simulink model "sliding"  (R2024a)
settings: Solver=FixedStepAuto  StartTime=0.0  StopTime=20  FixedStep=0.002  MaxStep=0.05  RelTol=1e-3
settings Model: Creator=Lenovo  LastModifiedBy=Lenovo
settings DebuggingCC: UnconnectedInputMsg=warning  UnconnectedOutputMsg=warning  UnconnectedLineMsg=warning
settings ModelReferenceCC: EnableRefExpFcnMdlSchedulingChecks=on
settings RTWCC: GPUComputeCapability=3.5  DLArmComputeVersion=19.05

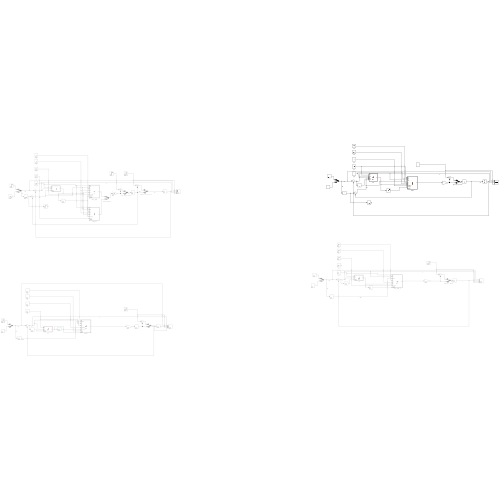
[thumbnail: Simulink's stored preview of the top-level diagram]
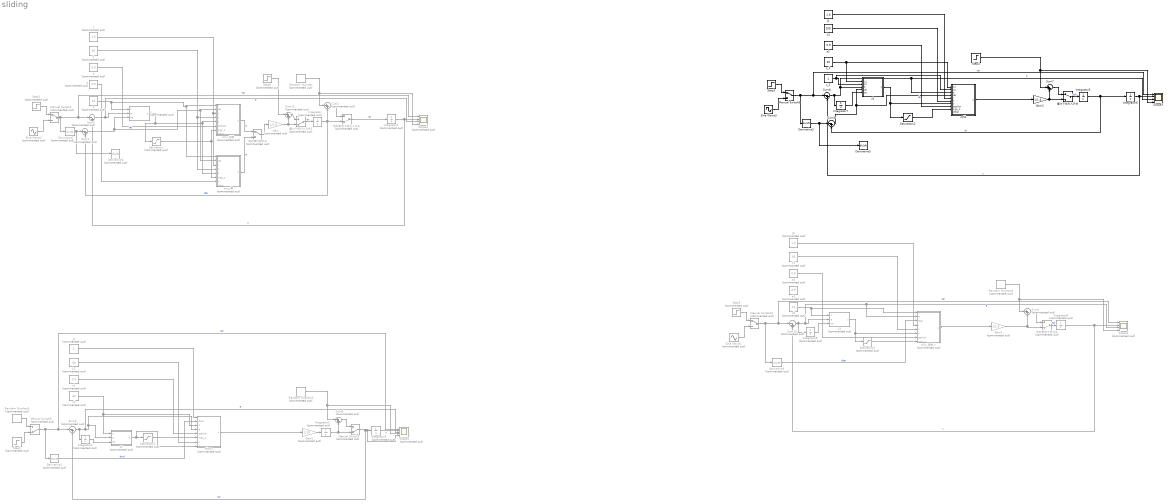
== system sliding ==
  Derivative{1..2,4,6} (4 alike) : Derivative  Commented=on
  Derivative3 : Derivative
  Derivative5 : Derivative
  Gain : Gain  Commented=on  Gain=1/1.6
  Gain1 : Gain  Commented=on  Gain=1/10
  Gain2 : Gain  Gain=1/1.6
  Gain3 : Gain  Commented=on  Gain=1/1.6
  Integrator{,1..4,8..9} (7 alike) : Integrator  Commented=on
  Integrator5 : Integrator
  Integrator6 : Integrator
  Integrator7 : Integrator
  J : Constant  Commented=on  Value=1.6
  J1 : Constant  Commented=on
  J2 : Constant  Value=1.6
  J3 : Constant  Commented=on  Value=1.6
  Manual Switch10 : ManualSwitch  Commented=on
  Manual Switch2 : ManualSwitch  Commented=on
  Manual Switch5 : ManualSwitch  Commented=on  CurrentSetting=0
  Manual Switch6 : ManualSwitch  Commented=on  CurrentSetting=0
  Manual Switch8 : ManualSwitch
  Random Number : RandomNumber  Commented=on  Seed=1  SampleTime=1
  Random Number2 : RandomNumber  Commented=on  Seed=1  SampleTime=1
  Random Number3 : RandomNumber  Commented=on  Variance=2  SampleTime=0.006
  Random Number4 : RandomNumber  Commented=on  Seed=1  SampleTime=1
  Saturation : Saturate  Commented=on  UpperLimit=0  LowerLimit=0
  Saturation1 : Saturate  Commented=on  UpperLimit=0  LowerLimit=0
  Saturation2 : Saturate  UpperLimit=0  LowerLimit=0
  Saturation3 : Saturate  Commented=on  UpperLimit=0  LowerLimit=0
  Scope1 : Scope  Commented=on  NumInputPorts=4
  Scope2 : Scope  Commented=on  NumInputPorts=5
  Scope3 : Scope  NumInputPorts=4
  Scope4 : Scope  Commented=on  NumInputPorts=4
  Sine Wave1 : Sin  Commented=on  Frequency=1*pi  SampleTime=0
  Sine Wave2 : Sin  Commented=on  Frequency=1*pi  SampleTime=0
  Sine Wave3 : Sin  Frequency=100*pi  SampleTime=0
  Step1 : Step  Commented=on  After=10  SampleTime=0
  Step2 : Step  Commented=on  SampleTime=0
  Step3 : Step  SampleTime=0
  Step4 : Step  After=50  SampleTime=0
  Step5 : Step  Commented=on  SampleTime=0
  Step6 : Step  Commented=on  After=50  SampleTime=0
  Sum{1..2,5,11} (4 alike) : Sum  Commented=on  Inputs=|++
  Sum{3..4,6,10} (4 alike) : Sum  Commented=on  Inputs=|-+
  Sum7 : Sum  Inputs=|++
  Sum8 : Sum  Inputs=|-+
  Sum9 : Sum  Inputs=|-+
  a : Constant  Commented=on  Value=0.9
  a1 : Constant  Commented=on  Value=0.9
  c : Constant  Commented=on  Value=13
  c1 : Constant  Commented=on  Value=40
  c2 : Constant  Commented=on  Value=13
  c_1 : Constant  Value=20
  c_2 : Constant
  ctrl4 : MATLAB Function  TreatAsAtomicUnit=on
  k : Constant  Commented=on  Value=95
  k1 : Constant  Commented=on  Value=60
  k2 : Constant  Value=200
  k3 : Constant  Commented=on  Value=95
  s : MATLAB Function  Commented=on  TreatAsAtomicUnit=on
  s1 : MATLAB Function  Commented=on  TreatAsAtomicUnit=on
  s2 : MATLAB Function  TreatAsAtomicUnit=on
  s3 : MATLAB Function  Commented=on  TreatAsAtomicUnit=on
  smc_幂 : MATLAB Function  Commented=on  TreatAsAtomicUnit=on
  smc_指数 : MATLAB Function  Commented=on  TreatAsAtomicUnit=on
  smc_指数_v : MATLAB Function  Commented=on  TreatAsAtomicUnit=on
  tfsmc : MATLAB Function  Commented=on  TreatAsAtomicUnit=on
  ε : Constant  Commented=on  Value=0.9
  ε1 : Constant  Commented=on  Value=0.5
  ε2 : Constant  Value=0.9
  ε3 : Constant  Commented=on  Value=0.8
  电机电流干扰开关 : ManualSwitch  Commented=on  CurrentSetting=0
  电机电流干扰引入开关 : ManualSwitch  Commented=on  CurrentSetting=0
  趋近律切换开关 : ManualSwitch  Commented=on
  重力干扰引入开关 : ManualSwitch
  重力干扰引入开关1 : ManualSwitch  Commented=on  CurrentSetting=0
  wires:
  c/1 -> smc_幂/1(c), smc_指数/1(c), s/1(c)
  Sum4/1 -> smc_幂/2(de), smc_指数/2(de), s/3(de)  "de"
  s/1(s) -> smc_幂/5(s), smc_指数/5(s), Saturation/1
  k/1 -> smc_幂/4(k), smc_指数/4(k)
  Step2/1 -> Manual Switch2/1
  Sine Wave2/1 -> Manual Switch2/2
  Integrator1/1 -> Scope1/2, Sum3/2  "x"
  J/1 -> smc_幂/3(J), smc_指数/3(J)
  ε/1 -> smc_指数/6(epsilon)
  Manual Switch2/1 -> Scope1/1, Sum3/1, Derivative2/1  "tar"
  Sum3/1 -> Scope1/3, s/2(e)  "e"
  Random Number/1 -> Scope1/4, Sum2/1
  Sum2/1 -> 电机电流干扰引入开关/1
  Integrator/1 -> Sum2/2, Sum4/2, 电机电流干扰引入开关/2  "ddx"
  smc_指数/1(u) -> 趋近律切换开关/1  "e"
  smc_幂/1(u) -> 趋近律切换开关/2  "e"
  趋近律切换开关/1 -> Gain/1
  Saturation/1 -> smc_指数/7(sign_s), smc_幂/6(sign_s)
  a/1 -> smc_幂/7(a)
  Sum5/1 -> Manual Switch5/1
  Random Number3/1 -> Manual Switch6/1
  Manual Switch6/1 -> Scope2/1, Sum6/1, Derivative1/1  "tar"
  Step1/1 -> Manual Switch6/2
  Sum6/1 -> Integrator4/1, Scope2/3, tfsmc/4(e), s1/2(e)  "e"
  Gain1/1 -> Integrator2/1
  Integrator2/1 -> Manual Switch5/2, Sum5/2
  c1/1 -> tfsmc/3(c), s1/1(c)
  tfsmc/1(u) -> Gain1/1
  Integrator3/1 -> Scope2/2  "x"
  Manual Switch5/1 -> Scope2/5, Integrator3/1, Sum6/2  "tar"
  Random Number2/1 -> Sum5/1, Scope2/4
  s1/1(s) -> tfsmc/8(s), Saturation1/1
  Integrator4/1 -> s1/3(se)
  Derivative1/1 -> tfsmc/2(dwd)  "dwd"
  Saturation1/1 -> tfsmc/6(sign_s)
  ε1/1 -> tfsmc/5(epsilon)
  J1/1 -> tfsmc/1(J)
  k1/1 -> tfsmc/7(k)
  Sum9/1 -> s2/4(de), ctrl4/4(de)  "de"
  Step4/1 -> Scope3/4, Sum7/1
  Manual Switch8/1 -> Scope3/1, Sum8/1, Derivative3/1  "tar"
  c_2/1 -> ctrl4/2(c2), s2/2(c2)
  Sine Wave3/1 -> Manual Switch8/2
  Integrator5/1 -> Sum9/2, Integrator6/1  "dx"
  k2/1 -> ctrl4/6(k)
  Step3/1 -> Manual Switch8/1
  ε2/1 -> ctrl4/8(epsilon)
  Integrator6/1 -> Scope3/2, Sum8/2  "x"
  Saturation2/1 -> ctrl4/9(sign_s)
  s2/1(s) -> Saturation2/1, ctrl4/7(s)
  J2/1 -> ctrl4/5(J)
  Sum7/1 -> 重力干扰引入开关/1
  ctrl4/1(u) -> Gain2/1
  Sum8/1 -> Integrator7/1, ctrl4/3(e), Scope3/3, s2/3(e)  "e"
  Integrator7/1 -> s2/5(se)
  c_1/1 -> s2/1(c1), ctrl4/1(c1)
  Derivative2/1 -> Derivative4/1, Sum4/1
  电机电流干扰引入开关/1 -> Integrator1/1  "dx"
  Gain2/1 -> 重力干扰引入开关/2, Sum7/2
  重力干扰引入开关/1 -> Integrator5/1  "ddx"
  Derivative3/1 -> Derivative5/1, Sum9/1
  电机电流干扰开关/1 -> Integrator8/1  "tar"
  Gain3/1 -> Sum1/2, 电机电流干扰开关/2
  Derivative6/1 -> smc_指数_v/3(dtar)  "dtar"
  k3/1 -> smc_指数_v/5(k)
  Sine Wave1/1 -> Manual Switch10/2
  ε3/1 -> smc_指数_v/7(epsilon)
  Saturation3/1 -> smc_指数_v/8(sign_s)
  c2/1 -> smc_指数_v/1(c), s3/1(c)
  Manual Switch10/1 -> Scope4/1, Sum10/1, Derivative6/1  "tar"
  Sum10/1 -> Integrator9/1, smc_指数_v/2(e), Scope4/3, s3/2(e)  "e"
  Integrator8/1 -> Scope4/2, Sum10/2  "v"
  s3/1(s) -> smc_指数_v/6(s), Saturation3/1
  J3/1 -> smc_指数_v/4(J)
  Sum1/1 -> 电机电流干扰开关/1
  smc_指数_v/1(u) -> Gain3/1
  Step5/1 -> Manual Switch10/1
  Random Number4/1 -> Scope4/4, Sum1/1
  Gain/1 -> Sum11/2, 重力干扰引入开关1/2
  Integrator9/1 -> s3/3(se)
  Step6/1 -> Sum11/1
  重力干扰引入开关1/1 -> Integrator/1  "dx"
  Sum11/1 -> 重力干扰引入开关1/1

== matlab function sliding/s2 ==
  data: c1 input; c2 input; s output; e input; de input; se input
function s = fcn(c1,c2,e,de,se)

s = c1*e+de+c2*se;

== matlab function sliding/smc_指数_v ==
  data: c input; e input; u output; dtar input; J input; k input; s input; epsilon input; sign_s input
function u = fcn(c,e,dtar,J,k,s,epsilon,sign_s)

u = J*(dtar - c*e - (k*s+epsilon*sign_s));

== matlab function sliding/smc_指数 ==
  data: c input; u output; de input; J input; k input; s input; epsilon input; sign_s input; ddtar input
function u = fcn(c,de,J,k,s,epsilon,sign_s,ddtar)

u = J*(-c*de + ddtar - (k*s+epsilon*sign_s));

== matlab function sliding/s3 ==
  data: c input; s output; e input; se input
function s = fcn(c,e,se)

s = e + c*se;

== matlab function sliding/smc_幂 ==
  data: c input; u output; de input; J input; k input; s input; sign_s input; a input; ddtar input
function u = fcn(c,de,J,k,s,sign_s,a,ddtar)

u = J*(-c*de + ddtar - k*s-k*(abs(s)^a)*sign_s);

== matlab function sliding/s ==
  data: c input; s output; e input; de input
function s = fcn(c,e,de)

s = c*e+de;

== matlab function sliding/tfsmc ==
  data: J input; dwd input; c input; e input; epsilon input; sign_s input; u output; k input; s input
function u = fcn(J,dwd,c,e,epsilon,sign_s,k,s)

u = J*(dwd-c*e-epsilon*sign_s-k*s);

== matlab function sliding/s1 ==
  data: c input; s output; e input; se input
function s = fcn(c,e,se)

s = e+c*se;

== matlab function sliding/ctrl4 ==
  data: c1 input; c2 input; e input; u output; de input; J input; k input; s input; epsilon input; sign_s input; ddtar input
function u = fcn(c1,c2,e,de,J,k,s,epsilon,sign_s,ddtar)

u = J*(-c1*de -c2*e + ddtar - (k*s+epsilon*sign_s));
